simulink model "DBO_of_inversekinermatics_of_xArm6DOF"  (R2021b)
settings: Solver=VariableStepAuto  StartTime=0.0  StopTime=10.0  RelTol=1e-3  AbsTol=1e-3  EnableMultiTasking=on
values from neighbouring files (symbols this model uses):
  B = [0; 0; 0; 0]    [InverseSolver_MDH.m]
  X = Pos(1)    [InverseSolver_MDH.m]
  Y = Pos(2)    [InverseSolver_MDH.m]
  Z = Pos(3)    [InverseSolver_MDH.m]
undefined symbols (not defined in the file or in its folder): Levenberg, Marquardt, Spline
libraries: sm_lib x24, nesl_utility x19, robotcorelib x4, robotmaniplib x3
settings Model: Creator=Sine  LastModifiedBy=Sine
settings SolverCC: AutoScaleAbsTol=off  AlgebraicLoopSolver=TrustRegion
settings DataIOCC: LimitDataPoints=on  MaxDataPoints=10000
settings OptimizationCC: LifeSpan=inf
settings DebuggingCC: AllowSymbolicDim=off  SFUnexpectedBacktrackingDiag=warning  SFNoUnconditionalDefaultTransitionDiag=warning  SFExecutionAtInitializationDiag=none  SFMachineParentedDataDiag=warning  ArithmeticOperatorsInVariantConditions=warning
settings SFSimCC: SimUseLocalCustomCode=off  CustomCodeUndefinedFunction=UseInterfaceOnly
settings RTWCC: RTWUseLocalCustomCode=off
settings CodeAppCC: StateflowObjectComments=on
settings GRTTargetCC: TargetLangStandard=C89/C90 (ANSI)
settings ConfigComp: CovMetricSettings=dw  CovSaveCumulativeToWorkspaceVar=on  CovSaveSingleToWorkspaceVar=on  CovExternalEMLEnable=off  CovSFcnEnable=off
settings SimscapeCC: SimscapeLogType=all  SimscapeLogSimulationStatistics=on  SimscapeLogDataHistory=10000

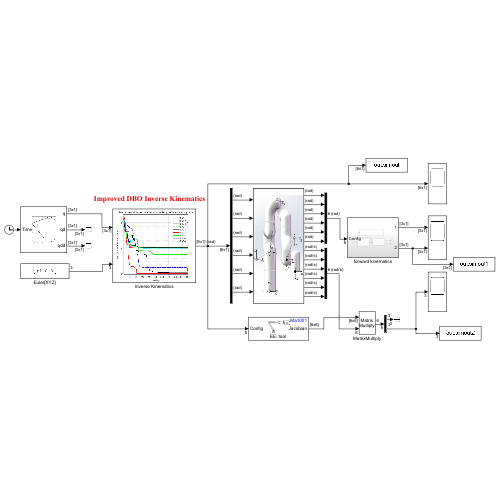
[thumbnail: Simulink's stored preview of the top-level diagram]
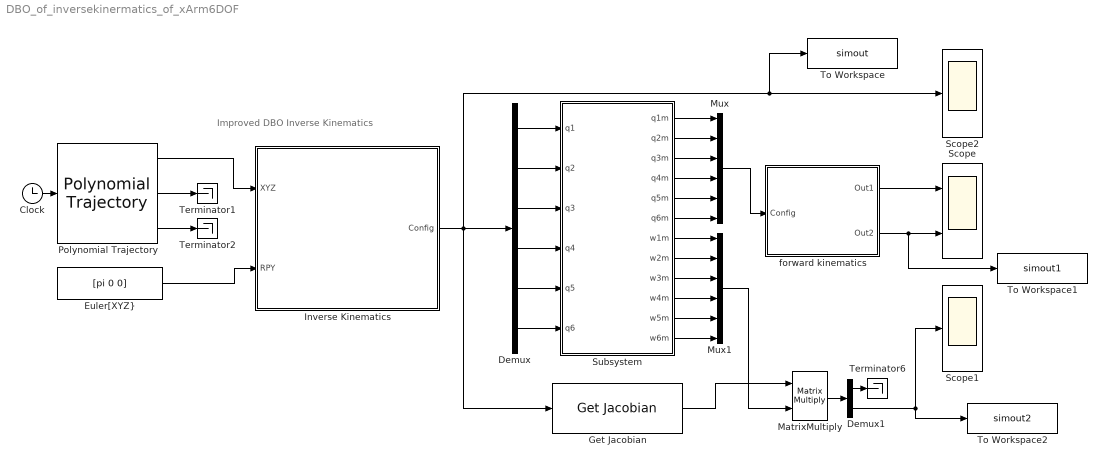
== system DBO_of_inversekinermatics_of_xArm6DOF ==
  note: Improved DBO Inverse Kinematics
  Clock : Clock
      settings: Decimation=60
  Demux : Demux  Outputs=6
  Demux1 : Demux  Outputs=2
  "Euler[XYZ}" : Constant  Value=[pi 0 0]
  Get Jacobian : robotmaniplib/Get Jacobian  RigidBodyTree=Ma1001  EndEffector=tool  SimulateUsing=Interpreted execution
      settings: SourceProductBaseCode=RO
  Inverse Kinematics : Subsystem
      mask Display: image('F:\Matlab\算法\Dung beetle optimize\robot-ik\Improved\idbo4.jpg'); % 使用工具条上的 "编辑图像" 进行更改。
  MatrixMultiply : Product  Multiplication=Matrix(*)
  Mux : Mux  Inputs=6
  Mux1 : Mux  Inputs=6
  Polynomial Trajectory : robotcorelib/Polynomial Trajectory  WaypointSource=Internal  Waypoints=P  TimePoints=N  TimeInterval=[ 0, 10 ]  Method=B-Spline  ParameterSource=Internal  VelocityBoundaryCondition=zeros( 3, 61 )  AccelerationBoundaryCondition=zeros( 2, 5 )  SimulateUsing=Interpreted execution
  Scope : Scope  NumInputPorts=2
  Scope1 : Scope
  Scope2 : Scope
  Subsystem : Subsystem
      mask Display: image('C:\Users\Sine\Desktop\Paper：robot inverse kinematic\xArm.jpg'); % 使用工具条上的 "编辑图像" 进行更改。
  Terminator1 : Terminator
  Terminator2 : Terminator
  Terminator6 : Terminator
  To Workspace : ToWorkspace  VariableName=simout  SampleTime=-1
  To Workspace1 : ToWorkspace  VariableName=simout1  SampleTime=-1
  To Workspace2 : ToWorkspace  VariableName=simout2  SampleTime=-1
  forward kinematics : Subsystem
  wires:
  Subsystem/1(q1m) -> Mux/1
  Subsystem/2(q2m) -> Mux/2
  Subsystem/3(q3m) -> Mux/3
  Subsystem/4(q4m) -> Mux/4
  Subsystem/5(q5m) -> Mux/5
  Subsystem/6(q6m) -> Mux/6
  Mux/1 -> forward kinematics/1(Config)
  Demux/1 -> Subsystem/1(q1)
  Demux/2 -> Subsystem/2(q2)
  Demux/3 -> Subsystem/3(q3)
  Demux/4 -> Subsystem/4(q4)
  Demux/5 -> Subsystem/5(q5)
  Demux/6 -> Subsystem/6(q6)
  Subsystem/7(w1m) -> Mux1/1
  Subsystem/8(w2m) -> Mux1/2
  Subsystem/9(w3m) -> Mux1/3
  Subsystem/10(w4m) -> Mux1/4
  Subsystem/11(w5m) -> Mux1/5
  Subsystem/12(w6m) -> Mux1/6
  Get Jacobian/1 -> MatrixMultiply/1
  Mux1/1 -> MatrixMultiply/2
  MatrixMultiply/1 -> Demux1/1
  Demux1/1 -> Terminator6/1
  Clock/1 -> Polynomial Trajectory/1
  Polynomial Trajectory/3 -> Terminator2/1
  Demux1/2 -> Scope1/1, To Workspace2/1
  Inverse Kinematics/1(Config) -> To Workspace/1, Scope2/1, Get Jacobian/1, Demux/1
  Polynomial Trajectory/1 -> Inverse Kinematics/1(XYZ)
  "Euler[XYZ}"/1 -> Inverse Kinematics/2(RPY)
  forward kinematics/1(Out1) -> Scope/1
  forward kinematics/2(Out2) -> To Workspace1/1, Scope/2
  Polynomial Trajectory/2 -> Terminator1/1

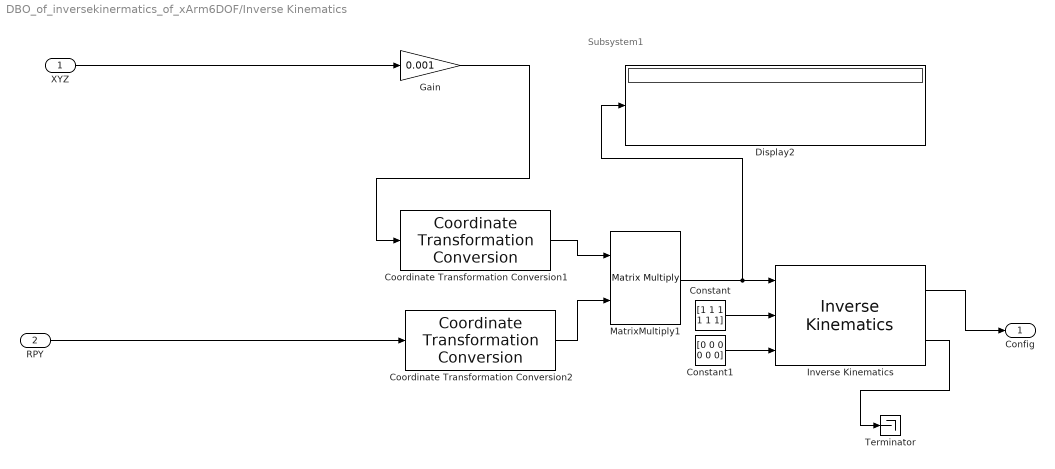
== system DBO_of_inversekinermatics_of_xArm6DOF/Inverse Kinematics ==
  note: Subsystem1
  XYZ : Inport
  RPY : Inport  Port=2
  Constant : Constant  Value=[1 1 1 1 1 1]
  Constant1 : Constant  Value=[0 0 0 0 0 0]
  Coordinate Transformation Conversion1 : robotcorelib/Coordinate Transformation Conversion  InputRepresentation=Translation Vector  InputEulerSequence=XYZ  ShowTrVecInputPort=off  OutputRepresentation=Homogeneous Transformation  OutputEulerSequence=ZYX  ShowTrVecOutputPort=on  SimulateUsing=Interpreted execution
      settings: SourceProductBaseCode=NV,RO,RR,UV
  Coordinate Transformation Conversion2 : robotcorelib/Coordinate Transformation Conversion  InputRepresentation=Euler Angles  InputEulerSequence=XYZ  ShowTrVecInputPort=off  OutputRepresentation=Homogeneous Transformation  OutputEulerSequence=ZYX  ShowTrVecOutputPort=on  SimulateUsing=Interpreted execution
      settings: SourceProductBaseCode=NV,RO,RR,UV
  Display2 : Display
  Gain : Gain  Gain=0.001
  Inverse Kinematics : robotmaniplib/Inverse Kinematics  RigidBodyTree=Ma1001  EndEffector=tool  ShowInfo=on  SolverName=Levenberg-Marquardt  EnforceJointLimits=on  MaxIterations=1500  MaxTime=10  GradientTolerance=1e-2  SolutionTolerance=1e-2  StepTolerance=1e-3  ErrorChangeTolerance=1e-3  UseErrorDamping=on  DampingBias=0.0025  SimulateUsing=Interpreted execution
  MatrixMultiply1 : Product  Multiplication=Matrix(*)
  Terminator : Terminator
  Config : Outport
  wires:
  Gain/1 -> Coordinate Transformation Conversion1/1
  Inverse Kinematics/2 -> Terminator/1
  Coordinate Transformation Conversion1/1 -> MatrixMultiply1/1
  MatrixMultiply1/1 -> Inverse Kinematics/1, Display2/1
  Coordinate Transformation Conversion2/1 -> MatrixMultiply1/2
  Constant1/1 -> Inverse Kinematics/3
  Constant/1 -> Inverse Kinematics/2
  RPY/1 -> Coordinate Transformation Conversion2/1
  Inverse Kinematics/1 -> Config/1
  XYZ/1 -> Gain/1

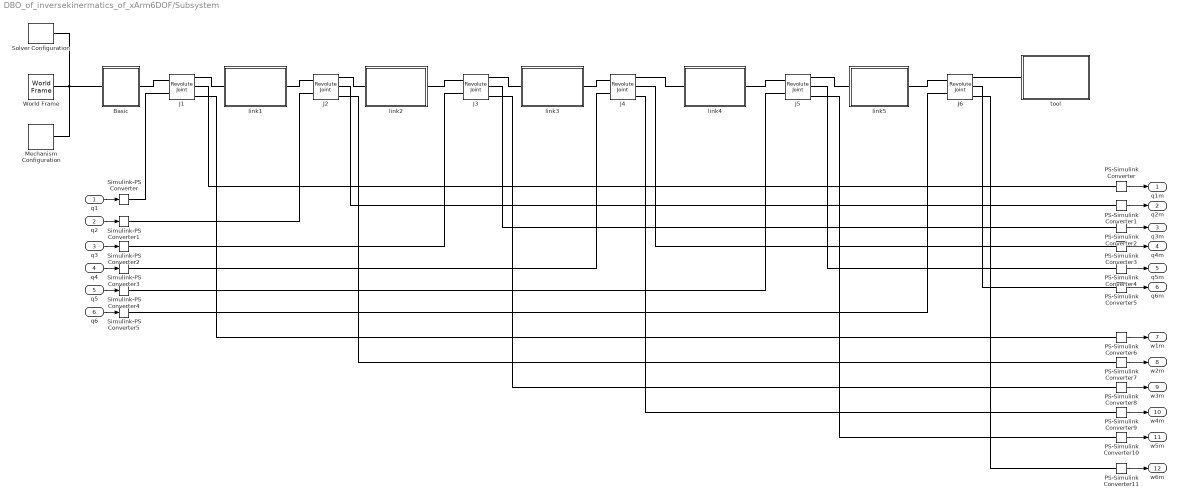
== system DBO_of_inversekinermatics_of_xArm6DOF/Subsystem ==
  q1 : Inport
  q2 : Inport  Port=2
  q3 : Inport  Port=3
  q4 : Inport  Port=4
  q5 : Inport  Port=5
  q6 : Inport  Port=6
  Basic : Subsystem
  J{1..6} (6 alike) : sm_lib/Joints/Revolute Joint  JointMode=Normal  SenseConstraintForce=off  SenseConstraintForceX=off  SenseConstraintForceY=off  SenseConstraintForceZ=off  SenseConstraintTorque=off  SenseConstraintTorqueX=off  SenseConstraintTorqueY=off  SenseConstraintTorqueZ=off  SenseTotalForce=off  SenseTotalForceX=off  SenseTotalForceY=off  SenseTotalForceZ=off  SenseTotalTorque=off  SenseTotalTorqueX=off  SenseTotalTorqueY=off  SenseTotalTorqueZ=off  CompositeWrenchDir=FollowerOnBase  CompositeWrenchFrame=BaseFrame  EquilibriumPosition=0  EquilibriumPositionUnits=deg  SpringStiffness=0  SpringStiffnessUnits=N*m/deg  DampingCoefficient=0  DampingCoefficientUnits=N*m/(deg/s)  TorqueActuationMode=ComputedTorque  MotionActuationMode=InputMotion  SensePosition=on  SenseVelocity=on  SenseAcceleration=off  SenseTorqueForce=off  SenseLowerLimitTorqueForce=off  SenseUpperLimitTorqueForce=off  LowerLimitSpecify=on  LowerLimitBound=-90  LowerLimitBoundUnits=deg  LowerLimitStiffness=1e4  LowerLimitStiffnessUnits=N*m/deg  LowerLimitDamping=10  LowerLimitDampingUnits=N*m/(deg/s)  LowerLimitTransitionRegionWidth=0.1  LowerLimitTransitionRegionWidthUnits=deg  UpperLimitSpecify=on  UpperLimitBound=90  UpperLimitBoundUnits=deg  UpperLimitStiffness=1e4  UpperLimitStiffnessUnits=N*m/deg  UpperLimitDamping=10  UpperLimitDampingUnits=N*m/(deg/s)  UpperLimitTransitionRegionWidth=0.1  UpperLimitTransitionRegionWidthUnits=deg  PositionTargetSpecify=off  PositionTargetPriority=High  PositionTargetValue=0  PositionTargetValueUnits=deg  VelocityTargetSpecify=off  VelocityTargetPriority=High  VelocityTargetValue=0  VelocityTargetValueUnits=deg/s
  Mechanism Configuration : sm_lib/Utilities/Mechanism Configuration  UniformGravity=Constant  GravityVector=[0 0 -9.80665]  GravityUnits=m/s^2  LinearizationDelta=0.001  JointModeTransitionNonlinearIterations=2
  PS-Simulink Converter{,1..11} (12 alike) : nesl_utility/PS-Simulink Converter  PhysicalDomain=network_engine_domain  SubClassName=ps_output  LeftPortType=input  RightPortType=output  PseudoPeriodic=off  Frequencies=[]  Unit=inherit  AffineConversion=off
      settings: SourceProductBaseCode=PW,SS
  Simulink-PS Converter{,1..5} (6 alike) : nesl_utility/Simulink-PS Converter  PhysicalDomain=network_engine_domain  SubClassName=ps_input  LeftPortType=input  RightPortType=output  PseudoPeriodic=off  Frequencies=[]  NoiseDistribution=none  NoiseParameters=[]  Unit=rad  AffineConversion=off  FilteringAndDerivatives=filter  SimscapeFilterOrder=2  InputFilterTimeConstant=0.001  UdotUserProvided=0
      settings: SourceProductBaseCode=PW,SS
  Solver Configuration : nesl_utility/Solver Configuration  PhysicalDomain=network_engine_domain  SubClassName=solver  LeftPortType=input  RightPortType=generic  Tones=[]  Harmonics=[]  SimulateNoise=off  Profile=off  UseLocalSampling=off  EnableSwitchedLinearOptims=on  FrequencyDomain=off  UseCCode=off  RelTol=0.001  AbsTol=1e-06  MinStep=1e-09  ToWorkspace=off  RevertToSquareIcSolve=off  NumHomotopyIterations=100  PhasorMode=off  PhasorModeNumHarmonics=1  DoDC=off  ResidualTolerance=1e-09  UseLocalSolver=off  LocalSolverChoice=NE_BACKWARD_EULER_ADVANCER  LocalSolverSampleTime=0.001  DoFixedCost=off  MaxNonlinIter=3  MaxModeIter=2  ComputeImpulses=off  ImpulseIterations=2  LinearAlgebra=Sparse  EquationFormulation=NE_TIME_EF  DelaysMemoryBudget=1024  AutomaticFiltering=on  FilteringTimeConstant=0.001  PartitionStorageMethod=AS_NEEDED  PartitionMemoryBudget=1024  PartitionMethod=FAST
      settings: SourceProductBaseCode=PW,SS
  World Frame : sm_lib/Frames and Transforms/World Frame
  link1 : Subsystem
  link2 : Subsystem
  link3 : Subsystem
  link4 : Subsystem
  link5 : Subsystem
  tool : Subsystem
  q1m : Outport
  q2m : Outport  Port=2
  q3m : Outport  Port=3
  q4m : Outport  Port=4
  q5m : Outport  Port=5
  q6m : Outport  Port=6
  w1m : Outport  Port=7
  w2m : Outport  Port=8
  w3m : Outport  Port=9
  w4m : Outport  Port=10
  w5m : Outport  Port=11
  w6m : Outport  Port=12
  wires:
  PS-Simulink Converter2/1 -> q3m/1
  q6/1 -> Simulink-PS Converter5/1
  q5/1 -> Simulink-PS Converter4/1
  PS-Simulink Converter4/1 -> q5m/1
  PS-Simulink Converter3/1 -> q4m/1
  PS-Simulink Converter/1 -> q1m/1
  q4/1 -> Simulink-PS Converter3/1
  q1/1 -> Simulink-PS Converter/1
  q2/1 -> Simulink-PS Converter1/1
  PS-Simulink Converter1/1 -> q2m/1
  PS-Simulink Converter5/1 -> q6m/1
  q3/1 -> Simulink-PS Converter2/1
  PS-Simulink Converter6/1 -> w1m/1
  PS-Simulink Converter7/1 -> w2m/1
  PS-Simulink Converter8/1 -> w3m/1
  PS-Simulink Converter9/1 -> w4m/1
  PS-Simulink Converter10/1 -> w5m/1
  PS-Simulink Converter11/1 -> w6m/1
  connections:
  PS-Simulink Converter5/LConn1 -- J6/RConn2
  Simulink-PS Converter/RConn1 -- J1/LConn2
  link1/LConn1 -- J1/RConn1
  World Frame/RConn1 -- Mechanism Configuration/RConn1 -- Basic/LConn1 -- Solver Configuration/RConn1
  Simulink-PS Converter5/RConn1 -- J6/LConn2
  PS-Simulink Converter4/LConn1 -- J5/RConn2
  PS-Simulink Converter3/LConn1 -- J4/RConn2
  PS-Simulink Converter/LConn1 -- J1/RConn2
  J1/LConn1 -- Basic/RConn1
  Simulink-PS Converter2/RConn1 -- J3/LConn2
  PS-Simulink Converter2/LConn1 -- J3/RConn2
  Simulink-PS Converter3/RConn1 -- J4/LConn2
  Simulink-PS Converter1/RConn1 -- J2/LConn2
  J2/RConn1 -- link2/LConn1
  Simulink-PS Converter4/RConn1 -- J5/LConn2
  J3/LConn1 -- link2/RConn1
  J6/LConn1 -- link5/RConn1
  link5/LConn1 -- J5/RConn1
  PS-Simulink Converter1/LConn1 -- J2/RConn2
  link4/LConn1 -- J4/RConn1
  J2/LConn1 -- link1/RConn1
  J5/LConn1 -- link4/RConn1
  link3/LConn1 -- J3/RConn1
  J4/LConn1 -- link3/RConn1
  J1/RConn3 -- PS-Simulink Converter6/LConn1
  J2/RConn3 -- PS-Simulink Converter7/LConn1
  J3/RConn3 -- PS-Simulink Converter8/LConn1
  J4/RConn3 -- PS-Simulink Converter9/LConn1
  J5/RConn3 -- PS-Simulink Converter10/LConn1
  J6/RConn3 -- PS-Simulink Converter11/LConn1
  tool/LConn1 -- J6/RConn1

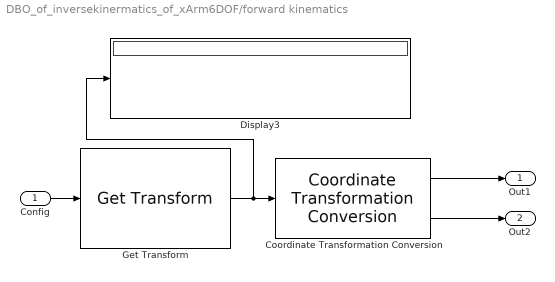
== system DBO_of_inversekinermatics_of_xArm6DOF/forward kinematics ==
  Config : Inport
  Coordinate Transformation Conversion : robotcorelib/Coordinate Transformation Conversion  InputRepresentation=Homogeneous Transformation  InputEulerSequence=ZYX  ShowTrVecInputPort=on  OutputRepresentation=Euler Angles  OutputEulerSequence=ZYX  ShowTrVecOutputPort=on  SimulateUsing=Interpreted execution
      settings: SourceProductBaseCode=NV,RO,RR,UV
  Display3 : Display
  Get Transform : robotmaniplib/Get Transform  RigidBodyTree=Ma1001  SourceBody=base  TargetBody=tool  SimulateUsing=Interpreted execution
  Out1 : Outport
  Out2 : Outport  Port=2
  wires:
  Get Transform/1 -> Display3/1, Coordinate Transformation Conversion/1
  Coordinate Transformation Conversion/1 -> Out1/1
  Config/1 -> Get Transform/1
  Coordinate Transformation Conversion/2 -> Out2/1

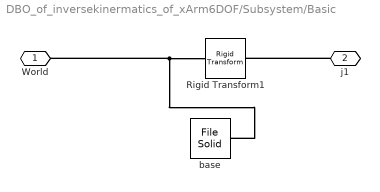
== system DBO_of_inversekinermatics_of_xArm6DOF/Subsystem/Basic ==
  Rigid Transform1 : sm_lib/Frames and Transforms/Rigid Transform  TranslationMethod=Cartesian  TranslationStandardOffset=154.8  TranslationLengthUnit=mm  TranslationStandardAxis=+Z  TranslationCartesianOffset=[0 0 154.8]  TranslationROffset=0  TranslationROffsetUnits=m  TranslationZOffset=0  TranslationZOffsetUnits=m  TranslationThetaOffset=0  TranslationThetaOffsetUnits=deg  RotationMethod=None  RotationAngleUnits=deg  RotationStandardAxis=+Z  RotationAngle=0.0  RotationArbitraryAxis=[0 0 1]  FollAlignAxisA=+X  BaseAlignAxisA=+Y  FollAlignAxisB=+Y  BaseAlignAxisB=+Z  RotationSequenceAxes=FollowerAxes  RotationSequence=XYX  RotationSequenceAngles=[0 0 0]  RotationSequenceAnglesUnits=deg  RotationMatrix=[1 0 0; 0 1 0; 0 0 1]
  base : sm_lib/Body Elements/File Solid  ExtGeomFileName=F:\Matlab\xArm6\x-t\J1.x_t  UnitType=FromFile  ExtGeomFileUnits=m  StepReaderType=HEX  ExportConvexHullGeometry=off  InertiaType=CalculateFromGeometry  Mass=3  MassUnits=kg  CenterOfMass=[0 0 0]  CenterOfMassUnits=m  MomentsOfInertia=[1 1 1]  MomentsOfInertiaUnits=kg*m^2  ProductsOfInertia=[0 0 0]  ProductsOfInertiaUnits=kg*m^2  BasedOnType=Mass  Density=1000  DensityUnits=kg/m^3  DoExposeReferenceFrame=on  SerializedFrames=<Frames/>  GraphicType=FromGeometry  MarkerShape=Sphere  MarkerSize=10  GraphicVisPropType=SimpleVisualProperties  GraphicDiffuseColor=[0.8 0.8 0.8]  GraphicSpecularColor=[0.5 0.5 0.5 1.0]  GraphicAmbientColor=[0.15 0.15 0.15 1.0]  GraphicEmissiveColor=[0.0 0.0 0.0 1.0]  GraphicShininess=75  GraphicOpacity=1.0
  World : PMIOPort  Side=Left
  j1 : PMIOPort  Port=2  Side=Right
  connections:
  base/RConn1 -- World/RConn1 -- Rigid Transform1/LConn1
  j1/RConn1 -- Rigid Transform1/RConn1

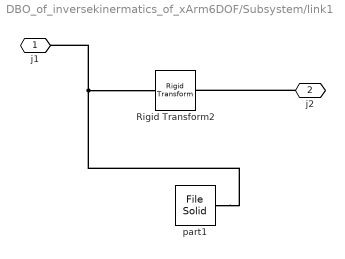
== system DBO_of_inversekinermatics_of_xArm6DOF/Subsystem/link1 ==
  Rigid Transform2 : sm_lib/Frames and Transforms/Rigid Transform  TranslationMethod=Cartesian  TranslationStandardOffset=112  TranslationLengthUnit=mm  TranslationStandardAxis=+Z  TranslationCartesianOffset=[0 112 75.32]  TranslationROffset=0  TranslationROffsetUnits=m  TranslationZOffset=0  TranslationZOffsetUnits=m  TranslationThetaOffset=0  TranslationThetaOffsetUnits=deg  RotationMethod=StandardAxis  RotationAngleUnits=deg  RotationStandardAxis=-X  RotationAngle=90  RotationArbitraryAxis=[0 0 1]  FollAlignAxisA=+X  BaseAlignAxisA=+Y  FollAlignAxisB=+Y  BaseAlignAxisB=+Z  RotationSequenceAxes=FollowerAxes  RotationSequence=XYX  RotationSequenceAngles=[0 0 0]  RotationSequenceAnglesUnits=deg  RotationMatrix=[1 0 0; 0 1 0; 0 0 1]
  part1 : sm_lib/Body Elements/File Solid  ExtGeomFileName=F:\Matlab\xArm6\x-t\J2.x_t  UnitType=FromFile  ExtGeomFileUnits=m  StepReaderType=HEX  ExportConvexHullGeometry=off  InertiaType=CalculateFromGeometry  Mass=2.177  MassUnits=kg  CenterOfMass=[0 0 0]  CenterOfMassUnits=m  MomentsOfInertia=[1 1 1]  MomentsOfInertiaUnits=kg*m^2  ProductsOfInertia=[0 0 0]  ProductsOfInertiaUnits=kg*m^2  BasedOnType=Mass  Density=1000  DensityUnits=kg/m^3  DoExposeReferenceFrame=on  SerializedFrames=<Frames/>  GraphicType=FromGeometry  MarkerShape=Sphere  MarkerSize=10  GraphicVisPropType=SimpleVisualProperties  GraphicDiffuseColor=[0.6 1.0 1.0]  GraphicSpecularColor=[0.5 0.5 0.5 1.0]  GraphicAmbientColor=[0.15 0.15 0.15 1.0]  GraphicEmissiveColor=[0.0 0.0 0.0 1.0]  GraphicShininess=75  GraphicOpacity=1.0
  j1 : PMIOPort  Side=Left
  j2 : PMIOPort  Port=2  Side=Right
  connections:
  part1/RConn1 -- j1/RConn1 -- Rigid Transform2/LConn1
  j2/RConn1 -- Rigid Transform2/RConn1

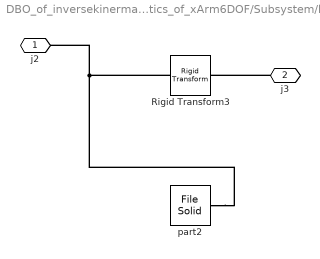
== system DBO_of_inversekinermatics_of_xArm6DOF/Subsystem/link2 ==
  Rigid Transform3 : sm_lib/Frames and Transforms/Rigid Transform  TranslationMethod=Cartesian  TranslationStandardOffset=112  TranslationLengthUnit=mm  TranslationStandardAxis=+Z  TranslationCartesianOffset=[53.96 -284.67 -8.3]  TranslationROffset=0  TranslationROffsetUnits=m  TranslationZOffset=0  TranslationZOffsetUnits=m  TranslationThetaOffset=0  TranslationThetaOffsetUnits=deg  RotationMethod=None  RotationAngleUnits=deg  RotationStandardAxis=-X  RotationAngle=90  RotationArbitraryAxis=[0 0 1]  FollAlignAxisA=+X  BaseAlignAxisA=+Y  FollAlignAxisB=+Y  BaseAlignAxisB=+Z  RotationSequenceAxes=FollowerAxes  RotationSequence=XYX  RotationSequenceAngles=[0 0 0]  RotationSequenceAnglesUnits=deg  RotationMatrix=[1 0 0; 0 1 0; 0 0 1]
  part2 : sm_lib/Body Elements/File Solid  ExtGeomFileName=F:\Matlab\xArm6\x-t\J3.x_t  UnitType=FromFile  ExtGeomFileUnits=m  StepReaderType=HEX  ExportConvexHullGeometry=off  InertiaType=CalculateFromGeometry  Mass=2.21  MassUnits=kg  CenterOfMass=[0 0 0]  CenterOfMassUnits=m  MomentsOfInertia=[1 1 1]  MomentsOfInertiaUnits=kg*m^2  ProductsOfInertia=[0 0 0]  ProductsOfInertiaUnits=kg*m^2  BasedOnType=Mass  Density=1000  DensityUnits=kg/m^3  DoExposeReferenceFrame=on  SerializedFrames=<Frames/>  GraphicType=FromGeometry  MarkerShape=Sphere  MarkerSize=10  GraphicVisPropType=SimpleVisualProperties  GraphicDiffuseColor=[0.6 0.6 1.0]  GraphicSpecularColor=[0.5 0.5 0.5 1.0]  GraphicAmbientColor=[0.15 0.15 0.15 1.0]  GraphicEmissiveColor=[0.0 0.0 0.0 1.0]  GraphicShininess=75  GraphicOpacity=1.0
  j2 : PMIOPort  Side=Left
  j3 : PMIOPort  Port=2  Side=Right
  connections:
  part2/RConn1 -- j2/RConn1 -- Rigid Transform3/LConn1
  j3/RConn1 -- Rigid Transform3/RConn1

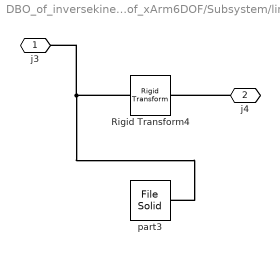
== system DBO_of_inversekinermatics_of_xArm6DOF/Subsystem/link3 ==
  Rigid Transform4 : sm_lib/Frames and Transforms/Rigid Transform  TranslationMethod=Cartesian  TranslationStandardOffset=67.19  TranslationLengthUnit=mm  TranslationStandardAxis=+X  TranslationCartesianOffset=[77.76 169.19 -67.49]  TranslationROffset=0  TranslationROffsetUnits=m  TranslationZOffset=0  TranslationZOffsetUnits=m  TranslationThetaOffset=0  TranslationThetaOffsetUnits=deg  RotationMethod=StandardAxis  RotationAngleUnits=deg  RotationStandardAxis=-X  RotationAngle=90  RotationArbitraryAxis=[0 0 1]  FollAlignAxisA=+X  BaseAlignAxisA=+Y  FollAlignAxisB=+Y  BaseAlignAxisB=+Z  RotationSequenceAxes=FollowerAxes  RotationSequence=XYX  RotationSequenceAngles=[0 0 0]  RotationSequenceAnglesUnits=deg  RotationMatrix=[1 0 0; 0 1 0; 0 0 1]
  part3 : sm_lib/Body Elements/File Solid  ExtGeomFileName=F:\Matlab\xArm6\x-t\J4.x_t  UnitType=FromFile  ExtGeomFileUnits=m  StepReaderType=HEX  ExportConvexHullGeometry=off  InertiaType=CalculateFromGeometry  Mass=1.925  MassUnits=kg  CenterOfMass=[0 0 0]  CenterOfMassUnits=m  MomentsOfInertia=[1 1 1]  MomentsOfInertiaUnits=kg*m^2  ProductsOfInertia=[0 0 0]  ProductsOfInertiaUnits=kg*m^2  BasedOnType=Mass  Density=1000  DensityUnits=kg/m^3  DoExposeReferenceFrame=on  SerializedFrames=<Frames/>  GraphicType=FromGeometry  MarkerShape=Sphere  MarkerSize=10  GraphicVisPropType=SimpleVisualProperties  GraphicDiffuseColor=[0.2 0.2 1.0]  GraphicSpecularColor=[0.5 0.5 0.5 1.0]  GraphicAmbientColor=[0.15 0.15 0.15 1.0]  GraphicEmissiveColor=[0.0 0.0 0.0 1.0]  GraphicShininess=75  GraphicOpacity=1.0
  j3 : PMIOPort  Side=Left
  j4 : PMIOPort  Port=2  Side=Right
  connections:
  Rigid Transform4/LConn1 -- part3/RConn1 -- j3/RConn1
  j4/RConn1 -- Rigid Transform4/RConn1

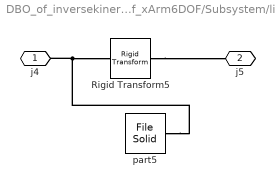
== system DBO_of_inversekinermatics_of_xArm6DOF/Subsystem/link4 ==
  Rigid Transform5 : sm_lib/Frames and Transforms/Rigid Transform  TranslationMethod=Cartesian  TranslationStandardOffset=-4.75  TranslationLengthUnit=mm  TranslationStandardAxis=+Y  TranslationCartesianOffset=[0 4.82 173]  TranslationROffset=0  TranslationROffsetUnits=m  TranslationZOffset=0  TranslationZOffsetUnits=m  TranslationThetaOffset=0  TranslationThetaOffsetUnits=deg  RotationMethod=StandardAxis  RotationAngleUnits=deg  RotationStandardAxis=+X  RotationAngle=90  RotationArbitraryAxis=[0 0 1]  FollAlignAxisA=+X  BaseAlignAxisA=+Y  FollAlignAxisB=+Y  BaseAlignAxisB=+Z  RotationSequenceAxes=FollowerAxes  RotationSequence=XYX  RotationSequenceAngles=[0 0 0]  RotationSequenceAnglesUnits=deg  RotationMatrix=[1 0 0; 0 1 0; 0 0 1]
  part5 : sm_lib/Body Elements/File Solid  ExtGeomFileName=F:\Matlab\xArm6\x-t\J5.x_t  UnitType=FromFile  ExtGeomFileUnits=m  StepReaderType=HEX  ExportConvexHullGeometry=off  InertiaType=CalculateFromGeometry  Mass=1.354  MassUnits=kg  CenterOfMass=[0 0 0]  CenterOfMassUnits=m  MomentsOfInertia=[1 1 1]  MomentsOfInertiaUnits=kg*m^2  ProductsOfInertia=[0 0 0]  ProductsOfInertiaUnits=kg*m^2  BasedOnType=Mass  Density=1000  DensityUnits=kg/m^3  DoExposeReferenceFrame=on  SerializedFrames=<Frames/>  GraphicType=FromGeometry  MarkerShape=Sphere  MarkerSize=10  GraphicVisPropType=SimpleVisualProperties  GraphicDiffuseColor=[0.8 0.8 1.0]  GraphicSpecularColor=[0.5 0.5 0.5 1.0]  GraphicAmbientColor=[0.15 0.15 0.15 1.0]  GraphicEmissiveColor=[0.0 0.0 0.0 1.0]  GraphicShininess=75  GraphicOpacity=1.0
  j4 : PMIOPort  Side=Left
  j5 : PMIOPort  Port=2  Side=Right
  connections:
  part5/RConn1 -- j4/RConn1 -- Rigid Transform5/LConn1
  Rigid Transform5/RConn1 -- j5/RConn1

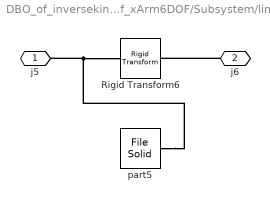
== system DBO_of_inversekinermatics_of_xArm6DOF/Subsystem/link5 ==
  Rigid Transform6 : sm_lib/Frames and Transforms/Rigid Transform  TranslationMethod=Cartesian  TranslationStandardOffset=-4.75  TranslationLengthUnit=mm  TranslationStandardAxis=+Y  TranslationCartesianOffset=[75.99 68.52 4.34]  TranslationROffset=0  TranslationROffsetUnits=m  TranslationZOffset=0  TranslationZOffsetUnits=m  TranslationThetaOffset=0  TranslationThetaOffsetUnits=deg  RotationMethod=StandardAxis  RotationAngleUnits=deg  RotationStandardAxis=-X  RotationAngle=90  RotationArbitraryAxis=[0 0 1]  FollAlignAxisA=+X  BaseAlignAxisA=+Y  FollAlignAxisB=+Y  BaseAlignAxisB=+Z  RotationSequenceAxes=FollowerAxes  RotationSequence=XYX  RotationSequenceAngles=[0 0 0]  RotationSequenceAnglesUnits=deg  RotationMatrix=[1 0 0; 0 1 0; 0 0 1]
  part5 : sm_lib/Body Elements/File Solid  ExtGeomFileName=F:\Matlab\xArm6\x-t\J6.x_t  UnitType=FromFile  ExtGeomFileUnits=m  StepReaderType=HEX  ExportConvexHullGeometry=off  InertiaType=CalculateFromGeometry  Mass=1.354  MassUnits=kg  CenterOfMass=[0 0 0]  CenterOfMassUnits=m  MomentsOfInertia=[1 1 1]  MomentsOfInertiaUnits=kg*m^2  ProductsOfInertia=[0 0 0]  ProductsOfInertiaUnits=kg*m^2  BasedOnType=Mass  Density=1000  DensityUnits=kg/m^3  DoExposeReferenceFrame=on  SerializedFrames=<Frames/>  GraphicType=FromGeometry  MarkerShape=Sphere  MarkerSize=10  GraphicVisPropType=SimpleVisualProperties  GraphicDiffuseColor=[0.6 0.6 1.0]  GraphicSpecularColor=[0.5 0.5 0.5 1.0]  GraphicAmbientColor=[0.15 0.15 0.15 1.0]  GraphicEmissiveColor=[0.0 0.0 0.0 1.0]  GraphicShininess=75  GraphicOpacity=1.0
  j5 : PMIOPort  Side=Left
  j6 : PMIOPort  Port=2  Side=Right
  connections:
  part5/RConn1 -- Rigid Transform6/LConn1 -- j5/RConn1
  j6/RConn1 -- Rigid Transform6/RConn1

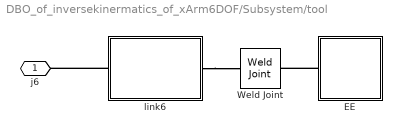
== system DBO_of_inversekinermatics_of_xArm6DOF/Subsystem/tool ==
  EE : Subsystem
  Weld Joint : sm_lib/Joints/Weld Joint  JointMode=Normal  SenseConstraintForce=off  SenseConstraintForceX=off  SenseConstraintForceY=off  SenseConstraintForceZ=off  SenseConstraintTorque=off  SenseConstraintTorqueX=off  SenseConstraintTorqueY=off  SenseConstraintTorqueZ=off  SenseTotalForce=off  SenseTotalForceX=off  SenseTotalForceY=off  SenseTotalForceZ=off  SenseTotalTorque=off  SenseTotalTorqueX=off  SenseTotalTorqueY=off  SenseTotalTorqueZ=off  CompositeWrenchDir=FollowerOnBase  CompositeWrenchFrame=BaseFrame
  link6 : Subsystem
  j6 : PMIOPort  Side=Left
  connections:
  EE/LConn1 -- Weld Joint/RConn1
  link6/RConn1 -- Weld Joint/LConn1
  link6/LConn1 -- j6/RConn1

== system DBO_of_inversekinermatics_of_xArm6DOF/Subsystem/tool/EE ==
  EE : sm_lib/Body Elements/File Solid  ExtGeomFileName=F:\Matlab\xArm6\x-t\End Effector.x_t  UnitType=FromFile  ExtGeomFileUnits=m  StepReaderType=HEX  ExportConvexHullGeometry=off  InertiaType=CalculateFromGeometry  Mass=0.55  MassUnits=kg  CenterOfMass=[0 0 0]  CenterOfMassUnits=m  MomentsOfInertia=[1 1 1]  MomentsOfInertiaUnits=kg*m^2  ProductsOfInertia=[0 0 0]  ProductsOfInertiaUnits=kg*m^2  BasedOnType=Mass  Density=1000  DensityUnits=kg/m^3  DoExposeReferenceFrame=on  SerializedFrames=<Frames/>  GraphicType=FromGeometry  MarkerShape=Sphere  MarkerSize=10  GraphicVisPropType=SimpleVisualProperties  GraphicDiffuseColor=[1.0 0.2 0.2]  GraphicSpecularColor=[0.5 0.5 0.5 1.0]  GraphicAmbientColor=[0.15 0.15 0.15 1.0]  GraphicEmissiveColor=[0.0 0.0 0.0 1.0]  GraphicShininess=75  GraphicOpacity=1.0
  Je : PMIOPort  Side=Left
  connections:
  EE/RConn1 -- Je/RConn1

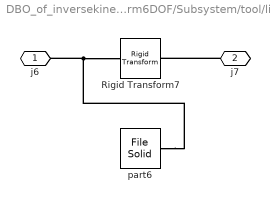
== system DBO_of_inversekinermatics_of_xArm6DOF/Subsystem/tool/link6 ==
  Rigid Transform7 : sm_lib/Frames and Transforms/Rigid Transform  TranslationMethod=Cartesian  TranslationStandardOffset=-4.75  TranslationLengthUnit=mm  TranslationStandardAxis=+Y  TranslationCartesianOffset=[0 0 28]  TranslationROffset=0  TranslationROffsetUnits=m  TranslationZOffset=0  TranslationZOffsetUnits=m  TranslationThetaOffset=0  TranslationThetaOffsetUnits=deg  RotationMethod=None  RotationAngleUnits=deg  RotationStandardAxis=+Z  RotationAngle=-90  RotationArbitraryAxis=[0 0 1]  FollAlignAxisA=+X  BaseAlignAxisA=+Y  FollAlignAxisB=+Y  BaseAlignAxisB=+Z  RotationSequenceAxes=FollowerAxes  RotationSequence=XYX  RotationSequenceAngles=[0 0 0]  RotationSequenceAnglesUnits=deg  RotationMatrix=[1 0 0; 0 1 0; 0 0 1]
  part6 : sm_lib/Body Elements/File Solid  ExtGeomFileName=F:\Matlab\xArm6\x-t\Tool head.x_t  UnitType=FromFile  ExtGeomFileUnits=m  StepReaderType=HEX  ExportConvexHullGeometry=off  InertiaType=CalculateFromGeometry  Mass=0.17  MassUnits=kg  CenterOfMass=[0 0 0]  CenterOfMassUnits=m  MomentsOfInertia=[1 1 1]  MomentsOfInertiaUnits=kg*m^2  ProductsOfInertia=[0 0 0]  ProductsOfInertiaUnits=kg*m^2  BasedOnType=Mass  Density=1000  DensityUnits=kg/m^3  DoExposeReferenceFrame=on  SerializedFrames=<Frames/>  GraphicType=FromGeometry  MarkerShape=Sphere  MarkerSize=10  GraphicVisPropType=SimpleVisualProperties  GraphicDiffuseColor=[0.4 0.0 1.0]  GraphicSpecularColor=[0.5 0.5 0.5 1.0]  GraphicAmbientColor=[0.15 0.15 0.15 1.0]  GraphicEmissiveColor=[0.0 0.0 0.0 1.0]  GraphicShininess=75  GraphicOpacity=1.0
  j6 : PMIOPort  Side=Left
  j7 : PMIOPort  Port=2  Side=Right
  connections:
  part6/RConn1 -- j6/RConn1 -- Rigid Transform7/LConn1
  j7/RConn1 -- Rigid Transform7/RConn1
